simulink model "sharedControlROS"  (R2018a)
settings: Solver=VariableStepAuto  StartTime=0.0  StopTime=500  RelTol=1e-3
values from neighbouring files (symbols this model uses):
  a = -real(s1) + imag(s1)/tan(angle(s1+b) - theta)    [RLDesignJoystick.m]
  a1 = b1/K    [RLDesignJoystick.m]
  a2 = 26.4940946148    [CrossTrackUSV.mat]
  b = 1.2*bb/I    (= 0.4)    [RLDesignJoystick.m]
  b1 = -real(s1)/150    [RLDesignJoystick.m]
  b2 = 0.266666666667    [CrossTrackUSV.mat]
  K0 = abs(s1+a)/abs(Gs1)/abs(s1+b)    [RLDesignJoystick.m]
  K1 = 1/abs(Gs1)    [RLDesignJoystick.m]
  K2 = 1619.40576956    [CrossTrackUSV.mat]
  U = 1.5    [CrossTrackUSV.mat]
libraries: robotlib x5, vrlib x1, sldrtlib x1, simulink x1
settings Model: Creator=KvonEllenrieder  LastModifiedBy=jrwam
settings CodeAppCC: StateflowObjectComments=on

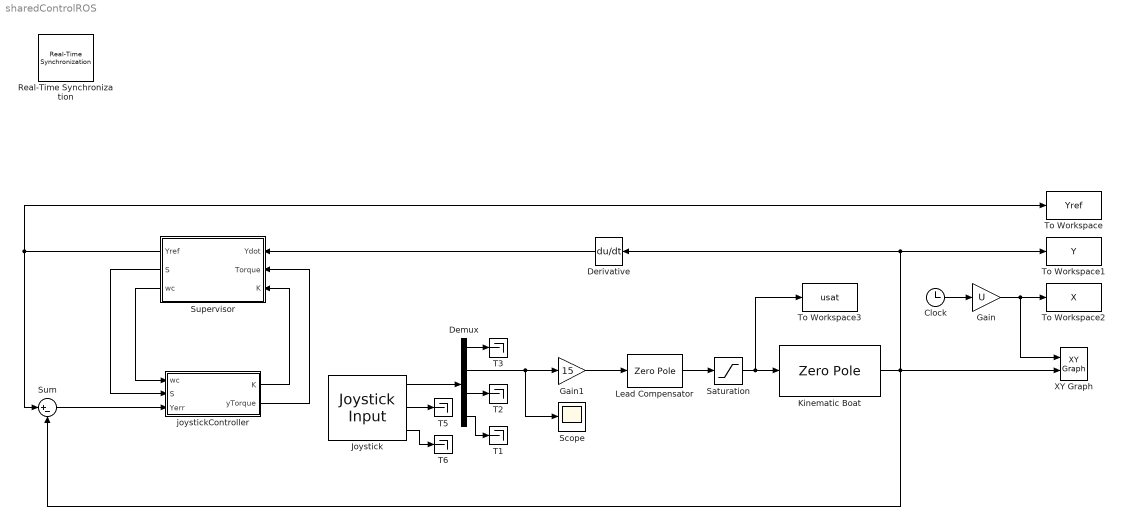
== system sharedControlROS ==
  Clock : Clock
  Demux : Demux
  Derivative : Derivative  CoefficientInTFapproximation=1
  Gain : Gain  Gain=U
  Gain1 : Gain  Gain=15
  Joystick : vrlib/Joystick Input  joyid=1  adjustports=on  forcefeed=off
      settings: SourceProductBaseCode=VR
  Kinematic Boat : ZeroPole  Zeros=[]  Poles=[0 0 -1.25]  Gain=[U*1e-2]
  Lead Compensator : ZeroPole  Zeros=[-b2]  Poles=[-a2]  Gain=[K2]
  Real-Time Synchronization : sldrtlib/Real-Time Synchronization  SampleTime=0.1  MaxMissedTicks=1000  ShowMissedTicks=off  YieldWhenWaiting=off
  Saturation : Saturate  UpperLimit=15  LowerLimit=-15
  Scope : Scope
  Sum : Sum  Inputs=|+-
  Supervisor : Subsystem
  T{1..3,5..6} (5 alike) : Terminator
  To Workspace : ToWorkspace  VariableName=Yref  SaveFormat=Timeseries  SampleTime=-1
  To Workspace1 : ToWorkspace  VariableName=Y  SaveFormat=Timeseries  SampleTime=-1
  To Workspace2 : ToWorkspace  VariableName=X  SaveFormat=Timeseries  SampleTime=-1
  To Workspace3 : ToWorkspace  VariableName=usat  SaveFormat=Timeseries  SampleTime=-1
  XY Graph : simulink/Sinks/XY Graph  xmin=-10  xmax=U*500  ymin=-7.5  ymax=7.5  st=-1
  joystickController : Subsystem
  wires:
  Lead Compensator/1 -> Saturation/1
  Saturation/1 -> Kinematic Boat/1, To Workspace3/1
  Clock/1 -> Gain/1
  Gain/1 -> To Workspace2/1, XY Graph/1
  Demux/4 -> T1/1
  Demux/3 -> T2/1
  Joystick/1 -> Demux/1
  Joystick/2 -> T5/1
  Joystick/3 -> T6/1
  Demux/1 -> T3/1
  Demux/2 -> Scope/1, Gain1/1
  Gain1/1 -> Lead Compensator/1
  Derivative/1 -> Supervisor/1(Ydot)
  Supervisor/1(Yref) -> Sum/1, To Workspace/1
  Kinematic Boat/1 -> XY Graph/2, Sum/2, To Workspace1/1, Derivative/1
  Sum/1 -> joystickController/3(Yerr)
  joystickController/2(yTorque) -> Supervisor/2(Torque)
  Supervisor/3(wc) -> joystickController/1(wc)
  joystickController/1(K) -> Supervisor/3(K)
  Supervisor/2(S) -> joystickController/2(S)

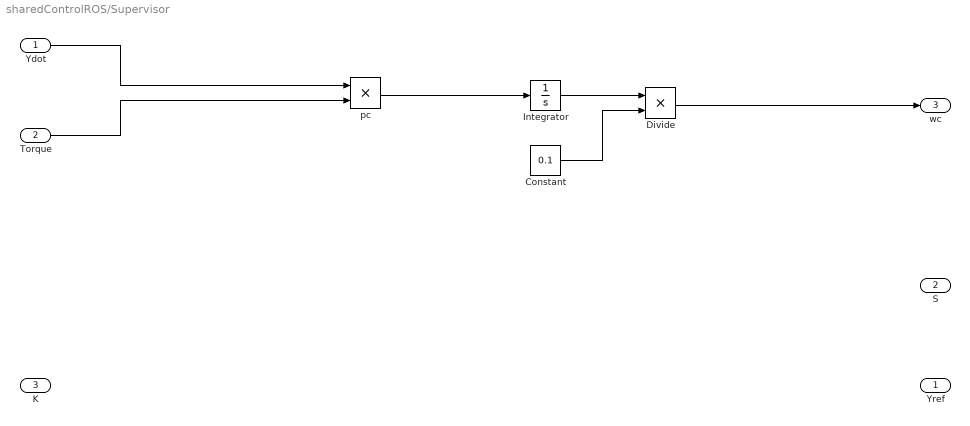
== system sharedControlROS/Supervisor ==
  Ydot : Inport
  Torque : Inport  Port=2
  K : Inport  Port=3
  Constant : Constant  Value=0.1
  Divide : Product
  Integrator : Integrator  ContinuousStateAttributes='wc'
  pc : Product
  Yref : Outport
  S : Outport  Port=2
  wc : Outport  Port=3
  wires:
  Ydot/1 -> pc/1
  Torque/1 -> pc/2
  pc/1 -> Integrator/1
  Integrator/1 -> Divide/1
  Constant/1 -> Divide/2
  Divide/1 -> wc/1

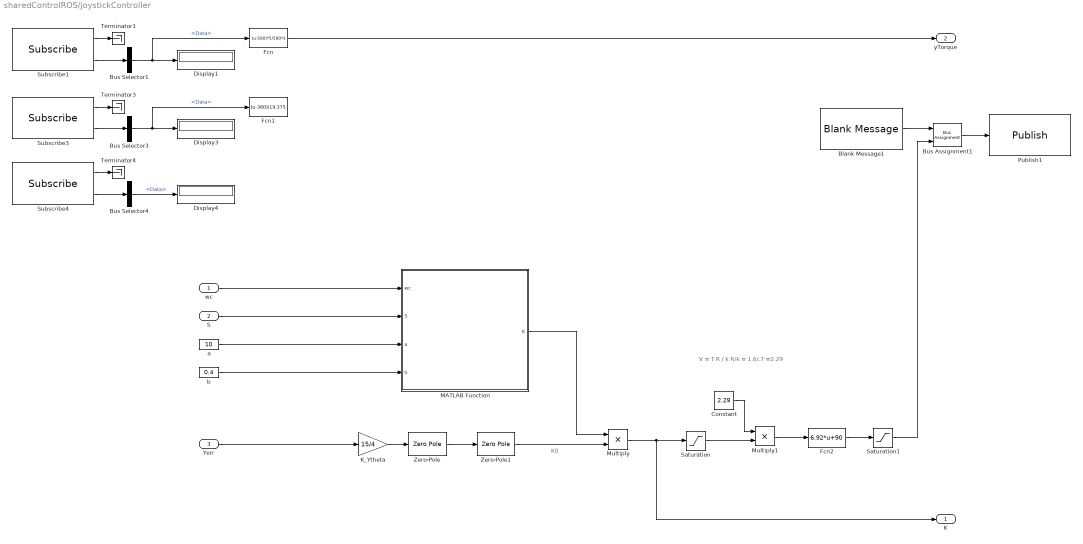
== system sharedControlROS/joystickController ==
  note: V = T R / k
      |
      | R/k = 1.6/.7 =2.29
  note: K0
  wc : Inport
  S : Inport  Port=2
  Yerr : Inport  Port=3
  Blank Message1 : robotlib/Blank Message  SourceLibraryInfo=This block requires Robotics System Toolbox  messageType=std_msgs/UInt16  SampleTime=inf
      settings: SourceProductBaseCode=RO
  Bus Assignment1 : BusAssignment  AssignedSignals=Data
  Bus Selector1 : BusSelector  OutputSignals=Data
  Bus Selector3 : BusSelector  OutputSignals=Data
  Bus Selector4 : BusSelector  OutputSignals=Data
  Constant : Constant  Value=2.29
  Display1 : Display
  Display3 : Display
  Display4 : Display
  Fcn : Fcn  Expr=(u-500)*5/500*3
  Fcn1 : Fcn  Expr=(u-380)/19.375
  Fcn2 : Fcn  Expr=6.92*u+90
  K_Ytheta : Gain  Gain=15/4
  MATLAB Function : MATLAB Function  TreatAsAtomicUnit=on
  Multiply : Product
  Multiply1 : Product
  Publish1 : robotlib/Publish  SourceLibraryInfo=This block requires Robotics System Toolbox  topicSource=Specify your own  topic=/yMotor  messageType=std_msgs/UInt16  messageQueueLength=1
      settings: SourceProductBaseCode=RO
  Saturation : Saturate  UpperLimit=3.5  LowerLimit=-3.5
  Saturation1 : Saturate  UpperLimit=180  LowerLimit=0
  Subscribe1 : robotlib/Subscribe  SourceLibraryInfo=This block requires Robotics System Toolbox  topicSource=Specify your own  topic=/yCurrent  messageType=std_msgs/UInt16  sampleTime=-1  messageQueueLength=1
      settings: SourceProductBaseCode=RO
  Subscribe3 : robotlib/Subscribe  SourceLibraryInfo=This block requires Robotics System Toolbox  topicSource=Specify your own  topic=/yPot  messageType=std_msgs/UInt16  sampleTime=-1  messageQueueLength=1
      settings: SourceProductBaseCode=RO
  Subscribe4 : robotlib/Subscribe  SourceLibraryInfo=This block requires Robotics System Toolbox  topicSource=Specify your own  topic=/debug  messageType=std_msgs/String  sampleTime=-1  messageQueueLength=1
      settings: SourceProductBaseCode=RO
  Terminator1 : Terminator
  Terminator3 : Terminator
  Terminator4 : Terminator
  Zero-Pole : ZeroPole  Zeros=[-b]  Poles=[-a]  Gain=[K0]
  Zero-Pole1 : ZeroPole  Zeros=[-b1]  Poles=[-a1]  Gain=[K1]
  a : Constant  Value=10
  b : Constant  Value=0.4
  K : Outport
  yTorque : Outport  Port=2
  wires:
  Blank Message1/1 -> Bus Assignment1/1
  Bus Assignment1/1 -> Publish1/1
  Bus Selector3/1 -> Fcn1/1, Display3/1  "<Data>"
  Fcn/1 -> yTorque/1
  Bus Selector4/1 -> Display4/1  "<Data>"
  Subscribe1/2 -> Bus Selector1/1
  Subscribe4/2 -> Bus Selector4/1
  Bus Selector1/1 -> Fcn/1, Display1/1  "<Data>"
  Subscribe3/2 -> Bus Selector3/1
  Subscribe3/1 -> Terminator3/1
  Subscribe1/1 -> Terminator1/1
  Subscribe4/1 -> Terminator4/1
  wc/1 -> MATLAB Function/1(wc)
  S/1 -> MATLAB Function/2(S)
  a/1 -> MATLAB Function/3(a)
  b/1 -> MATLAB Function/4(b)
  Yerr/1 -> K_Ytheta/1
  K_Ytheta/1 -> Zero-Pole/1
  Saturation/1 -> Multiply1/2
  Zero-Pole/1 -> Zero-Pole1/1
  Zero-Pole1/1 -> Multiply/2
  Multiply/1 -> K/1, Saturation/1
  MATLAB Function/1(K) -> Multiply/1
  Constant/1 -> Multiply1/1
  Multiply1/1 -> Fcn2/1
  Fcn2/1 -> Saturation1/1
  Saturation1/1 -> Bus Assignment1/2

== matlab function sharedControlROS/joystickController/MATLAB Function ==
  data: wc input; K output; S input; a input; b input
function K = fcn(wc, S, a, b)

if S == 2    
    K = 1/(1 + exp(-a*wc + b));
else
    K = 1;
end

return
